simulink model "sldemo_msfcn_lms"  (Simulink 7.6)
settings: Solver=FixedStepDiscrete  StartTime=0.0  StopTime=20000  FixedStep=0.1  RelTol=1e-3
PreLoadFcn:
  | b = [ -0.0012   -0.0014    0.0020    0.0029   -0.0044   -0.0064    0.0090    0.0125 -0.0169   -0.0227    0.0305    0.0412   -0.0573   -0.0850    0.1472    0.4501 0.4501    0.1472   -0.0850   -0.0573    0.0412    0.0305   -0.0227   -0.0169 0.0125    0.0090   -0.0064   -0.0044    0.0029    0.0020   -0.0014   -0.0012];
CloseFcn:
  | clear b
settings Model: Creator=The MathWorks Inc.  ExtModeAutoUpdateStatusClock=off
settings OptimizationCC: InlineInvariantSignals=on  InitFltsAndDblsToZero=on
settings DebuggingCC: SaveWithParameterizedLinksMsg=none  SignalResolutionControl=TryResolveAllWithWarning  MultiTaskDSMMsg=warning  MultiTaskCondExecSysMsg=none
settings RTWCC: IncludeERTFirstTime=on
settings GRTTargetCC: TargetFcnLib=ansi_tfl_tmw.mat

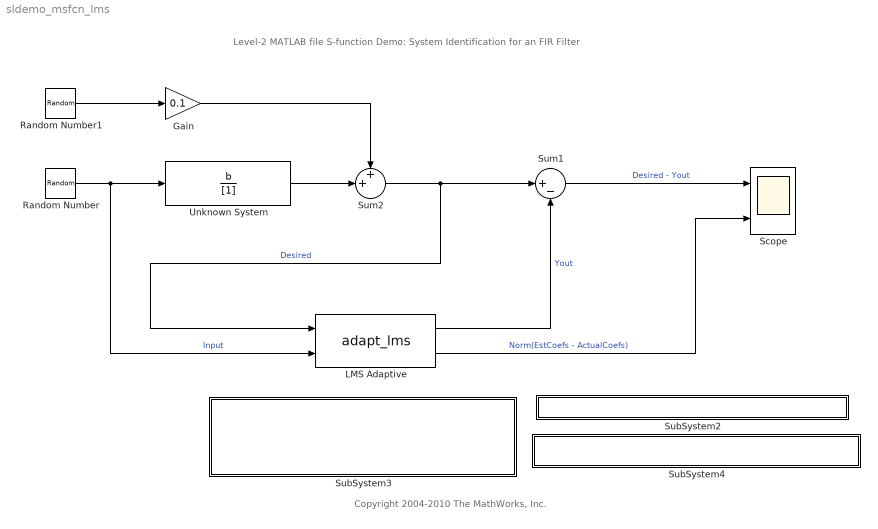
== system sldemo_msfcn_lms ==
  note: Level-2 MATLAB file S-function Demo:
      | System Identification for an FIR Filter
  note: Copyright 2004-2010 The MathWorks, Inc.
  Gain : Gain  Gain=0.1
  LMS Adaptive : M-S-Function  FunctionName=adapt_lms  Parameters=0.005
  Random Number : RandomNumber  SampleTime=1
  Random Number1 : RandomNumber  Seed=3  SampleTime=1
  Scope : Scope  NumInputPorts=2
      settings: TimeRange=2000  YMin=-1.5~0  YMax=1.5~0.7
  SubSystem2 : Subsystem
      settings: OpenFcn=edit(fullfile(matlabroot,'toolbox','simulink','simdemos','simfeatures','adapt_lms.tlc'))
      mask Display: disp('matlabroot\toolbox\simulink\simdemos\simfeatures\adapt_lms.tlc');
  SubSystem3 : Subsystem
      settings: OpenFcn=|
      | hFig = figure(1);
      | act = stem(b');
      | hold on;
      | est = stem(zeros(size(b')),'filled','r');
      | hold off;
      | tAxis  = findobj(hFig,'Type','axes');
      | tLines = findobj(tAxis(1),'Type','Line');
      | for i = 1:length(tLines)
      |   set(tLines(i), 'EraseMode', 'xor');
      | end
      | legend([act, est],'Actual','Estimated');
      | xlabel('Coefficient #');
      | ylabel('Coefficient Value');
      | grid on;
      | set_param('sldemo_msfcn_lms/LMS Adaptive','UserData',hFig);
      | add_adapt_coef_plot
      mask Display: disp('Double click here while simulation is running\n to add a PostOutputs event callback for \nplotting the current estimated filter coefficients.');
  SubSystem4 : Subsystem  mask{filename=adapt_lms.m}
      mask init:
      | x=sfundemo_maskdisp;
      settings: AttributesFormatString=\n  OpenFcn=sfundemo_openfcn
      mask Display: disp(x);
  Sum1 : Sum  Inputs=|+-
  Sum2 : Sum  Inputs=++|
  Unknown System : DiscreteFilter  Numerator=b  Denominator=[1]
  wires:
  Random Number/1 -> Unknown System/1, LMS Adaptive/2  "Input"
  Sum2/1 -> Sum1/1, LMS Adaptive/1  "Desired"
  Sum1/1 -> Scope/1  "Desired - Yout"
  Unknown System/1 -> Sum2/2
  LMS Adaptive/1 -> Sum1/2  "Yout"
  Gain/1 -> Sum2/1
  Random Number1/1 -> Gain/1
  LMS Adaptive/2 -> Scope/2  "Norm(EstCoefs - ActualCoefs)"

== system sldemo_msfcn_lms/SubSystem2 ==

== system sldemo_msfcn_lms/SubSystem3 ==

== system sldemo_msfcn_lms/SubSystem4 ==
